simulink model "Media_TtoT1_Converter"  (R2022b)
settings: Solver=VariableStepAuto  StartTime=0.0  StopTime=10.0  RelTol=1e-3
settings Model: DataDictionary=Optimate_PhysicalArchiDD.sldd  Creator=TO41629  LastModifiedBy=TO41629

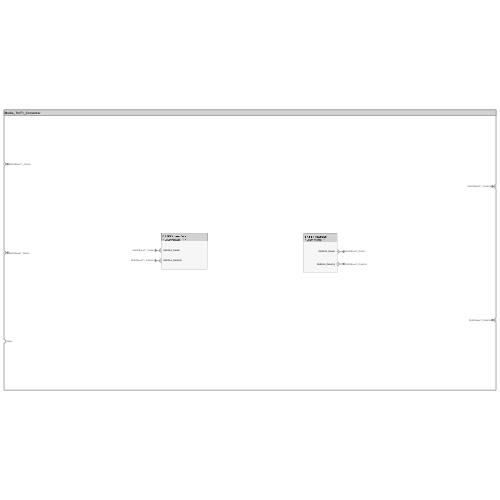
[thumbnail: Simulink's stored preview of the top-level diagram]
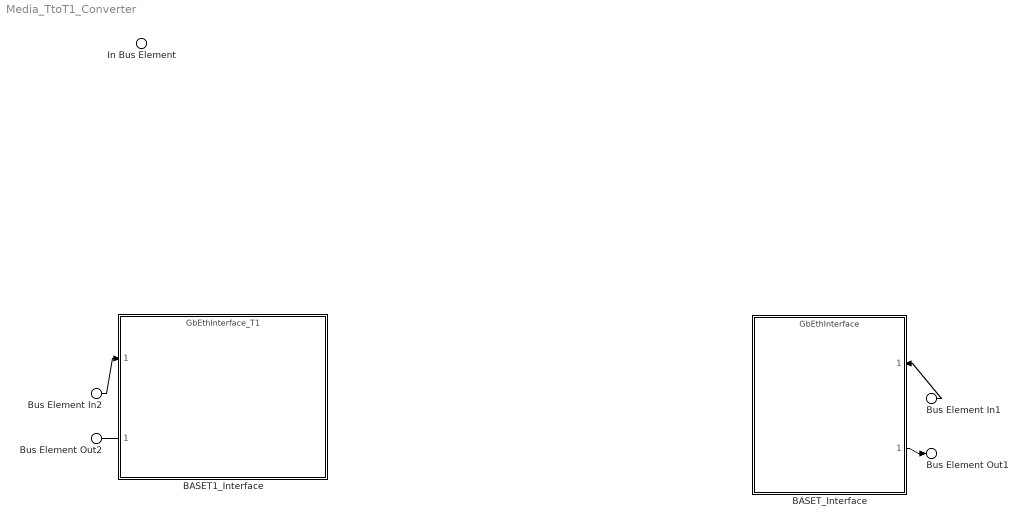
== system Media_TtoT1_Converter ==
  Bus Element In2 : Inport  PortName=GbEthBaseT1_DataIn
  Bus Element In1 : Inport  Port=2  PortName=GbEthBaseT_DataIn
  In Bus Element : Inport  Port=3  PortName=PowerSupply
  BASET1_Interface : ModelReference  ModelNameDialog=GbEthInterface_T1  UsingDefaultArgumentValue=0,0,0  SimulationMode=Normal  ModelReferenceVersion=1.29
      settings: PortSchema="{\"entries\":[{\"content\":{\"headerSize\":38,\"margin\":15,\"minimumSpacing\":25,\"sides\":[{\"content\":{\"connectorIds\":[\"In1\",\"Out1\"]},\"type\":\"ConnectorPlacement.EquallySpacedRectSide\",\"uuid\":\"99f9264f-b53d-4971-8b33-a510fd21d3a3\"},{\"content\":{\"connectorIds\":[],\"side\":\"RIGHT\"},\"type\":\"ConnectorPlacement.EquallySpacedRectSide\",\"uuid\":\"2d9ba29c-7f97-48cb-9608-186fea073d48\"},{\"content\":{\"connectorIds\":[],\"side\":\"TOP\"},\"type\":\"ConnectorPlacement.EquallySpacedRectSide\",\"uuid\":\"4aabfdd9-8cc9-4862-a428-8fddf83f7eb0\"}]},\"type\":\"ConnectorPlacement.EquallySpacedConnector\",\"uuid\":\"0c6b3b40-bc47-4abe-952f-60d13c7625c4\"}],\"packageUris\":[\"http://schema.mathworks.com/mf0/Connector/R2020b\"],\"version\":\"1.0\"}"
  BASET_Interface : ModelReference  ModelNameDialog=GbEthInterface  UsingDefaultArgumentValue=0,0,0  SimulationMode=Normal  ModelReferenceVersion=1.28
      settings: PortSchema="{\"entries\":[{\"content\":{\"headerSize\":38,\"margin\":15,\"minimumSpacing\":25,\"sides\":[{\"content\":{\"connectorIds\":[]},\"type\":\"ConnectorPlacement.EquallySpacedRectSide\",\"uuid\":\"99f9264f-b53d-4971-8b33-a510fd21d3a3\"},{\"content\":{\"connectorIds\":[\"In1\",\"Out1\"],\"side\":\"RIGHT\"},\"type\":\"ConnectorPlacement.EquallySpacedRectSide\",\"uuid\":\"2d9ba29c-7f97-48cb-9608-186fea073d48\"},{\"content\":{\"connectorIds\":[],\"side\":\"TOP\"},\"type\":\"ConnectorPlacement.EquallySpacedRectSide\",\"uuid\":\"4aabfdd9-8cc9-4862-a428-8fddf83f7eb0\"}]},\"type\":\"ConnectorPlacement.EquallySpacedConnector\",\"uuid\":\"0c6b3b40-bc47-4abe-952f-60d13c7625c4\"}],\"packageUris\":[\"http://schema.mathworks.com/mf0/Connector/R2020b\"],\"version\":\"1.0\"}"
  Bus Element Out2 : Outport  PortName=GbEthBaseT1_DataOut
  Bus Element Out1 : Outport  Port=2  PortName=GbEthBaseT_DataOut
  wires:
  Bus Element In1/1 -> BASET_Interface/1
  BASET_Interface/1 -> Bus Element Out1/1
  Bus Element In2/1 -> BASET1_Interface/1
  BASET1_Interface/1 -> Bus Element Out2/1
